simulink model "AWG"  (R2019a)
settings: Solver=FixedStepDiscrete  StartTime=0.0  StopTime=N_sim  RelTol=1e-3  EnableMultiTasking=on
PostLoadFcn:
  | AWG_Init
InitFcn:
  | %% DSPBuilder Start
  | alt_dspbuilder_update_model(bdroot)
  | %% DSPBuilder End
  | 
  | AWG_Init
StartFcn:
  | %% DSPBuilder Start
  | alt_dspbuilder_hdlimport_prepare_for_simulation(bdroot)
  | %% DSPBuilder End
StopFcn:
  | AWG_Analyse
values from neighbouring files (symbols this model uses):
  N_bits = 10    [AWG_Init.m]
  N_cnt = ceil(log2(MemSize))    [AWG_Init.m]
libraries: allblocks_alteradspbuilder2 x33, dspsrcs4 x3
settings Model: Creator=Kortke  LastModifiedBy=kortke
settings DataIOCC: LimitDataPoints=on  SaveFormat=Array  SignalLoggingSaveFormat=ModelDataLogs  ReturnWorkspaceOutputs=off
settings OptimizationCC: ExpressionDepthLimit=2147483647  InitFltsAndDblsToZero=on  LifeSpan=inf
settings DebuggingCC: UnderspecifiedInitializationDetection=Classic  MergeDetectMultiDrivingBlocksExec=none  SolverPrmCheckMsg=warning  FcnCallInpInsideContextMsg=warning  AllowSymbolicDim=off  StateNameClashWarn=warning  SFUnexpectedBacktrackingDiag=warning  SFNoUnconditionalDefaultTransitionDiag=warning  SFExecutionAtInitializationDiag=none  ArithmeticOperatorsInVariantConditions=warning
settings HardwareCC: ProdBitPerPointer=32  ProdBitPerSizeT=32  ProdBitPerPtrDiffT=32  ProdLargestAtomicFloat=None  ProdIntDivRoundTo=Undefined  ProdEndianess=Unspecified  ProdWordSize=32  ProdHWDeviceType=32-bit Generic
settings ModelReferenceCC: PropagateSignalLabelsOutOfModel=off
settings SFSimCC: SimUseLocalCustomCode=off
settings RTWCC: RTWUseLocalCustomCode=off
settings CodeAppCC: StateflowObjectComments=on
settings GRTTargetCC: TargetLangStandard=C89/C90 (ANSI)  CombineOutputUpdateFcns=off  GRTInterface=on
settings ConfigComp: CovMetricSettings=dw  CovHtmlReporting=on  CovSaveCumulativeToWorkspaceVar=on  CovSaveSingleToWorkspaceVar=on  CovExternalEMLEnable=off

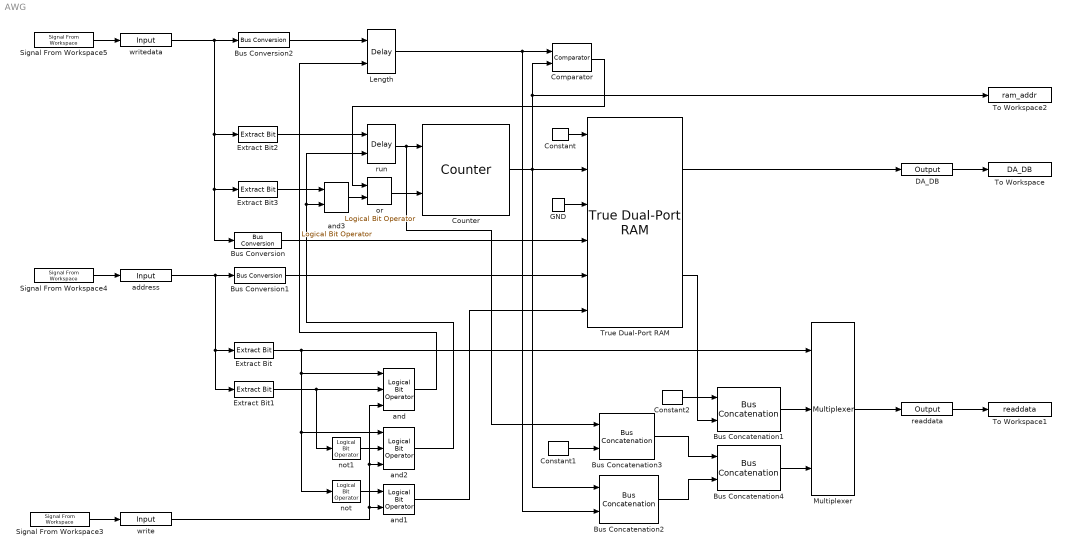
== system AWG ==
  Bus Concatenation1 : allblocks_alteradspbuilder2/Bus Concatenation  isSigned=off  awidth=32-N_bits  bwidth=N_bits  pipeline_display=0
  Bus Concatenation2 : allblocks_alteradspbuilder2/Bus Concatenation  isSigned=off  awidth=N_cnt  bwidth=N_cnt  pipeline_display=0
  Bus Concatenation3 : allblocks_alteradspbuilder2/Bus Concatenation  isSigned=off  awidth=1  bwidth=32-2*N_cnt-1  pipeline_display=0
  Bus Concatenation4 : allblocks_alteradspbuilder2/Bus Concatenation  isSigned=off  awidth=32-2*N_cnt  bwidth=2*N_cnt  pipeline_display=0
  Bus Conversion : allblocks_alteradspbuilder2/Bus Conversion  BusType=Signed Integer  ibwl=32  ibwr=1  bwl=N_bits  bwr=1  bitToConnectToOutputLSB=0  round=off  saturate=off  pipeline_display=0
  Bus Conversion1 : allblocks_alteradspbuilder2/Bus Conversion  BusType=Signed Integer  ibwl=N_cnt+1  ibwr=1  bwl=N_cnt  bwr=1  bitToConnectToOutputLSB=0  round=off  saturate=off  pipeline_display=0
  Bus Conversion2 : allblocks_alteradspbuilder2/Bus Conversion  BusType=Unsigned Integer  ibwl=32  ibwr=1  bwl=N_cnt  bwr=1  bitToConnectToOutputLSB=0  round=off  saturate=off  pipeline_display=0
  Comparator : allblocks_alteradspbuilder2/Comparator  direction=a == b  pipeline_display=0  allowFloatingPointOverride=on  logOutputs=off  logFile=D:\projects\Lehre\IDS\Projektbeispiele\AWG\tb_AWG\AWG_Comparator.fixedpointlog
  Constant : allblocks_alteradspbuilder2/Constant  mask_cst=0  BusType=Unsigned Integer  bwl=N_bits  bwr=0  roundMode=Truncate  satMode=Wrap  SpecifyClock=off  allowFloatingPointOverride=on  logOutputs=off  logFile=D:\projects\Lehre\IDS\Projektbeispiele\AWG\tb_AWG\AWG_Constant.fixedpointlog
  Constant1 : allblocks_alteradspbuilder2/Constant  mask_cst=0  BusType=Unsigned Integer  bwl=32-2*N_cnt-1  bwr=0  roundMode=Truncate  satMode=Wrap  SpecifyClock=off  allowFloatingPointOverride=on  logOutputs=off  logFile=D:\projects\Lehre\IDS\Projektbeispiele\AWG\tb_AWG\AWG_Constant1.fixedpointlog
  Constant2 : allblocks_alteradspbuilder2/Constant  mask_cst=0  BusType=Unsigned Integer  bwl=32-N_bits  bwr=0  roundMode=Truncate  satMode=Wrap  SpecifyClock=off  allowFloatingPointOverride=on  logOutputs=off  logFile=D:\projects\Lehre\IDS\Projektbeispiele\AWG\tb_AWG\AWG_Constant2.fixedpointlog
  Counter : allblocks_alteradspbuilder2/Counter  BusType=Unsigned Integer  bwl=N_cnt  bwr=0  use_modulo=off  modulo=255  SpecifyClock=off  direction=Increment  use_sload=off  use_sset=off  svalue=1  use_clk_ena=off  use_ena=on  use_sclr=on  pipeline_display=1
  DA_DB : allblocks_alteradspbuilder2/Output  iofile=D:\projects\Lehre\IDS\Projektbeispiele\AWG\tb_AWG\AWG_DA%5FDB.capture  BusType=Unsigned Integer  bwl=N_bits  bwr=0  externalType=Inferred  PORTTYPE=Output  allowFloatingPointOverride=on  logOutputs=off
  Extract Bit : allblocks_alteradspbuilder2/Extract Bit  BusType=Unsigned Integer  bwl=N_cnt+1  bwr=1  bitToSelect=N_cnt  pipeline_display=0
  Extract Bit1 : allblocks_alteradspbuilder2/Extract Bit  BusType=Unsigned Integer  bwl=N_cnt+1  bwr=1  bitToSelect=0  pipeline_display=0
  Extract Bit2 : allblocks_alteradspbuilder2/Extract Bit  BusType=Unsigned Integer  bwl=32  bwr=1  bitToSelect=0  pipeline_display=0
  Extract Bit3 : allblocks_alteradspbuilder2/Extract Bit  BusType=Unsigned Integer  bwl=32  bwr=1  bitToSelect=1  pipeline_display=0
  GND : allblocks_alteradspbuilder2/GND  SpecifyClock=off
  Length : allblocks_alteradspbuilder2/Delay  pipeline=1  pipeline_display=1  ClockPhase=1  use_ena=on  use_sclr=off  allowFloatingPointOverride=on  logOutputs=off  logFile=D:\projects\Lehre\IDS\Projektbeispiele\AWG\tb_AWG\AWG_Length.fixedpointlog  use_init=off  reset_value=1
  Multiplexer : allblocks_alteradspbuilder2/Multiplexer  numInputs=2  pipeline=1  oneHot=off  pipeline_display=1  use_ena=off  use_aclr=off  allowFloatingPointOverride=on  logOutputs=off  logFile=D:\projects\Lehre\IDS\Projektbeispiele\AWG\tb_AWG\AWG_Multiplexer.fixedpointlog
  Signal From Workspace3 : dspsrcs4/Signal From Workspace  X=write  Ts=1  nsamps=1  OutputAfterFinalValue=Setting to zero  ignoreOrWarnInputAndFrameLengths=off  OutputFrames=on
  Signal From Workspace4 : dspsrcs4/Signal From Workspace  X=address  Ts=1  nsamps=1  OutputAfterFinalValue=Setting to zero  ignoreOrWarnInputAndFrameLengths=off  OutputFrames=on
  Signal From Workspace5 : dspsrcs4/Signal From Workspace  X=writedata  Ts=1  nsamps=1  OutputAfterFinalValue=Setting to zero  ignoreOrWarnInputAndFrameLengths=off  OutputFrames=on
  To Workspace : ToWorkspace  VariableName=DA_DB  SampleTime=-1
      settings: Save2DSignal=2-D array (concatenate along first dimension)
  To Workspace1 : ToWorkspace  VariableName=readdata  SampleTime=-1
      settings: Save2DSignal=2-D array (concatenate along first dimension)
  To Workspace2 : ToWorkspace  VariableName=ram_addr  SampleTime=-1
      settings: Save2DSignal=2-D array (concatenate along first dimension)
  True Dual-Port RAM : allblocks_alteradspbuilder2/True Dual-Port RAM  numwords=MemSize  BusType=Unsigned Integer  bwl=N_bits  bwr=0  memory_type=AUTO  ram_type=TrueDualRAM  dont_care=off  initialization=Blank  init_file=input.hex  init_array=mem_data  register_outputs=off  use_ena=off  ClockPhase=1  pipeline_display=1  allowFloatingPointOverride=on  logOutputs=off  logFile=D:\projects\Lehre\IDS\Projektbeispiele\AWG\tb_AWG\AWG_True+Dual-Port+RAM%3A%3Aq%5Fa.fixedpointlog,D:\projects\Lehre\IDS\Projektbeispiele\AWG\tb_AWG\AWG_True+Dual-Port+RAM%3A%3Aq%5Fb.fixedpointlog,
  address : allblocks_alteradspbuilder2/Input  iofile=D:\projects\Lehre\IDS\Projektbeispiele\AWG\tb_AWG\AWG_address.salt  BusType=Unsigned Integer  bwl=N_cnt+1  bwr=0  SpecifyClock=off  PORTTYPE=Input  externalType=Inferred  allowFloatingPointOverride=on  logOutputs=off
  and : allblocks_alteradspbuilder2/Logical Bit Operator  LogicalOperator=AND  user_inputs=3  pipeline_display=0
  and1 : allblocks_alteradspbuilder2/Logical Bit Operator  LogicalOperator=AND  user_inputs=2  pipeline_display=0
  and2 : allblocks_alteradspbuilder2/Logical Bit Operator  LogicalOperator=AND  user_inputs=3  pipeline_display=0
  and3 : allblocks_alteradspbuilder2/Logical Bit Operator  LogicalOperator=AND  user_inputs=2  pipeline_display=0
  not : allblocks_alteradspbuilder2/Logical Bit Operator  LogicalOperator=NOT  user_inputs=2  pipeline_display=0
  not1 : allblocks_alteradspbuilder2/Logical Bit Operator  LogicalOperator=NOT  user_inputs=2  pipeline_display=0
  or : allblocks_alteradspbuilder2/Logical Bit Operator  LogicalOperator=OR  user_inputs=2  pipeline_display=0
  readdata : allblocks_alteradspbuilder2/Output  iofile=D:\projects\Lehre\IDS\Projektbeispiele\AWG\tb_AWG\AWG_readdata.capture  BusType=Unsigned Integer  bwl=32  bwr=0  externalType=Inferred  PORTTYPE=Output  allowFloatingPointOverride=on  logOutputs=off
  run : allblocks_alteradspbuilder2/Delay  pipeline=1  pipeline_display=1  ClockPhase=1  use_ena=on  use_sclr=off  allowFloatingPointOverride=on  logOutputs=off  logFile=D:\projects\Lehre\IDS\Projektbeispiele\AWG\tb_AWG\AWG_run.fixedpointlog  use_init=off  reset_value=1
  write : allblocks_alteradspbuilder2/Input  iofile=D:\projects\Lehre\IDS\Projektbeispiele\AWG\tb_AWG\AWG_write.salt  BusType=Single Bit  bwl=32  bwr=0  SpecifyClock=off  PORTTYPE=Input  externalType=Inferred  allowFloatingPointOverride=on  logOutputs=off
  writedata : allblocks_alteradspbuilder2/Input  iofile=D:\projects\Lehre\IDS\Projektbeispiele\AWG\tb_AWG\AWG_writedata.salt  BusType=Unsigned Integer  bwl=32  bwr=0  SpecifyClock=off  PORTTYPE=Input  externalType=Inferred  allowFloatingPointOverride=on  logOutputs=off
  wires:
  DA_DB/1 -> To Workspace/1
  Signal From Workspace4/1 -> address/1
  Signal From Workspace3/1 -> write/1
  Signal From Workspace5/1 -> writedata/1
  readdata/1 -> To Workspace1/1
  Constant/1 -> True Dual-Port RAM/1
  Bus Conversion/1 -> True Dual-Port RAM/4
  GND/1 -> True Dual-Port RAM/3
  Bus Conversion1/1 -> True Dual-Port RAM/5
  or/1 -> Counter/2
  Length/1 -> Comparator/1, Bus Concatenation2/2
  Bus Conversion2/1 -> Length/1
  Comparator/1 -> or/1
  write/1 -> and1/2, and2/3, and/3
  Extract Bit/1 -> Multiplexer/1, and/1, and2/1, not/1
  and1/1 -> True Dual-Port RAM/6
  Bus Concatenation1/1 -> Multiplexer/2
  True Dual-Port RAM/2 -> Bus Concatenation1/2
  Constant2/1 -> Bus Concatenation1/1
  Counter/1 -> Bus Concatenation2/1, To Workspace2/1, Comparator/2, True Dual-Port RAM/2
  True Dual-Port RAM/1 -> DA_DB/1
  Multiplexer/1 -> readdata/1
  writedata/1 -> Bus Conversion2/1, Extract Bit2/1, Bus Conversion/1, Extract Bit3/1
  address/1 -> Bus Conversion1/1, Extract Bit1/1, Extract Bit/1
  Extract Bit1/1 -> and/2, not1/1
  Extract Bit2/1 -> run/1
  and3/1 -> or/2
  Extract Bit3/1 -> and3/1
  not/1 -> and1/1
  not1/1 -> and2/2
  and/1 -> Length/2
  and2/1 -> and3/2, run/2
  Bus Concatenation4/1 -> Multiplexer/3
  Bus Concatenation2/1 -> Bus Concatenation4/2
  Bus Concatenation3/1 -> Bus Concatenation4/1
  Constant1/1 -> Bus Concatenation3/2
  run/1 -> Bus Concatenation3/1, Counter/1
